simulink model "tez_model_quadcopter1"  (R2021b)
settings: Solver=VariableStepAuto  StartTime=0  StopTime=20  FixedStep=10e-3  RelTol=1e-3
values from neighbouring files (symbols this model uses):
  b = 3.59 * 10^(-5)    (= 3.59e-05)    [LQR_controller.m]
  d = 2.081 * 10^(-6)    (= 2.081e-06)    [LQR_controller.m]
  g = 9.81    [LQR_controller.m]
  Ix = 0.00963    [LQR_controller.m]
  Iy = 0.00963    [LQR_controller.m]
  Iz = 0.019    [LQR_controller.m]
  Jr = 5.225 * 10^(-5)    (= 5.225e-05)    [LQR_controller.m]
  K = lqr(A,B,Q,R)    [LQR_controller.m]
  l = 0.24    [LQR_controller.m]
  m = 0.9928    [LQR_controller.m]
undefined symbols (not defined in the file or in its folder): rad, s, sigbuilder_block
libraries: simulink_extras x5, aerolibconvert2 x4, aerolibwind2 x2, aerolibnav x2, simulink x1, sensorgpslib x1, visionsinks x1, sim3dcameralib x1, sim3dlib x1, uavsim3dlib x1
settings Model: PacingRate=1000  Creator=sevba  LastModifiedBy=SEVBAN ALTAY
settings DataIOCC: SaveFormat=StructureWithTime
settings OptimizationCC: BlockReduction=off  BufferReuse=off  ZeroExternalMemoryAtStartup=off  ZeroInternalMemoryAtStartup=off
settings DebuggingCC: AlgebraicLoopMsg=none  UnconnectedInputMsg=none  UnconnectedOutputMsg=none  UnconnectedLineMsg=none
settings RTWCC: GenCodeOnly=on  TargetLang=C++
settings GRTTargetCC: TargetLangStandard=C++11 (ISO)  CodeInterfacePackaging=C++ class
settings ExplorerConfigSet: SimMechanicsOpenEditorOnUpdate=off

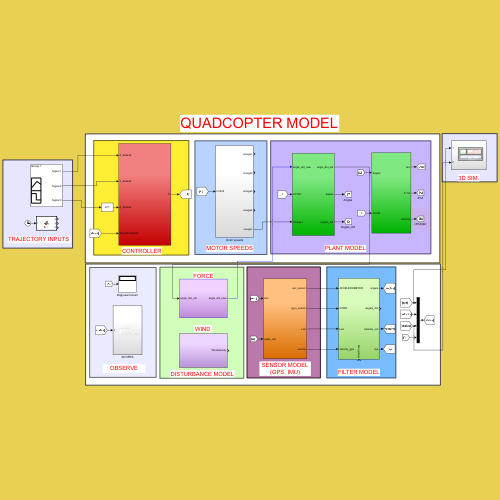
[thumbnail: Simulink's stored preview of the top-level diagram]
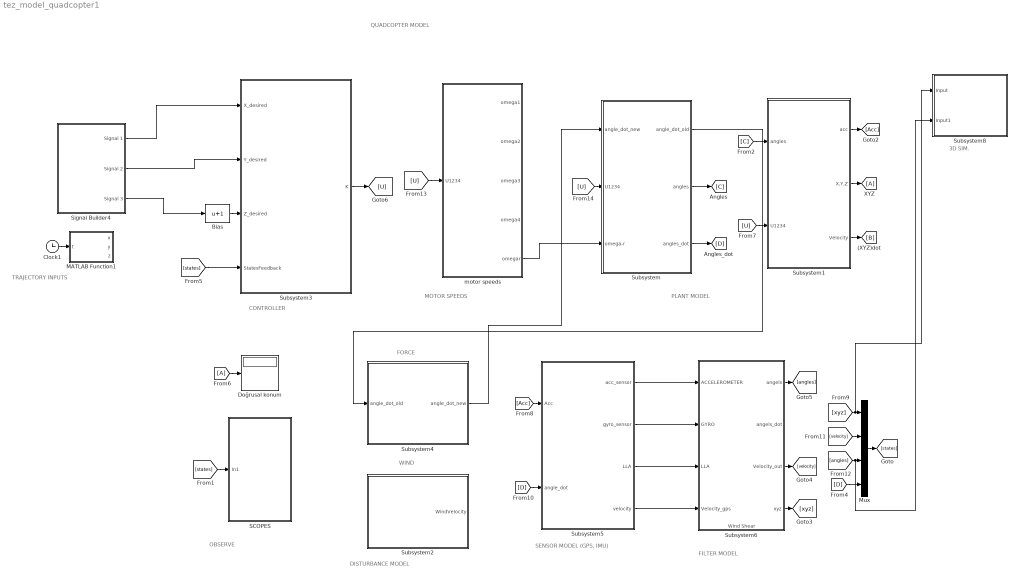
== system tez_model_quadcopter1 ==
  note: PLANT MODEL
  note: CONTROLLER
  note: MOTOR SPEEDS
  note: SENSOR MODEL
      | (GPS, IMU)
  note: FILTER MODEL
  note: DISTURBANCE MODEL
  note: OBSERVE
  note: QUADCOPTER MODEL
  note: FORCE
  note: WIND
  note: 3D SIM.
  note: TRAJECTORY INPUTS
  Bias : Bias  Bias=1
  Clock1 : Clock
  Doğrusal konum : Display
  MATLAB Function1 : MATLAB Function  TreatAsAtomicUnit=on
  Mux : Mux
  SCOPES : Subsystem
  Signal Builder4 : Subsystem  Tag=STV Subsys  LoadFcn=sigbuilder_block('load');  StartFcn=sigbuilder_block('start');  StopFcn=sigbuilder_block('stop');  ClipboardFcn=sigbuilder_block('clipboard');  mask(Sigbuilder block){tuvar=[0:10]}
      mask help: Simulink:masks:SigbuilderBlock_MD
      mask init:
      | if ~strcmp(get_param(bdroot(gcbh),'SimulationStatus'),'stopped') tuvar = sigbuilder_block('maskInit'); end
      settings: CopyFcn=sigbuilder_block('copy');  DeleteFcn=sigbuilder_block('delete');  ModelCloseFcn=sigbuilder_block('modelClose');  PreSaveFcn=sigbuilder_block('preSave');  PauseFcn=sigbuilder_block('pause');  ContinueFcn=sigbuilder_block('continue');  NameChangeFcn=sigbuilder_block('namechange');  OpenFcn=sigbuilder_block('open',[437.6 199.2 550.4 400 ]);  CloseFcn=sigbuilder_block('close');
      mask Display: plot(0, 0, 100, 100,[2, 2, 32, 32, 2], [68, 8, 8, 68, 68],[32, 2], [38, 38], [32, 19, 2],[53, 60, 44], [32, 17, 17, 2],[16, 16, 31, 31]);txt = getActiveGroup(gcbh);text(2, 100, txt,'verticalAlignment', 'top');
  Subsystem : Subsystem
  Subsystem1 : Subsystem
  Subsystem2 : Subsystem
  Subsystem3 : Subsystem
  Subsystem4 : Subsystem
  Subsystem5 : Subsystem
  Subsystem6 : Subsystem
      settings: PortSchema="{\"entries\":[{\"content\":{\"sides\":[{\"content\":{\"connectorIds\":[\"In1\",\"In2\",\"In3\",\"In4\"]},\"type\":\"ConnectorPlacement.EquallySpacedRectSide\",\"uuid\":\"cc522a2d-3ba1-4f01-ae64-adf2ce2f9772\"},{\"content\":{\"connectorIds\":[\"Out1\",\"Out2\",\"Out3\",\"Out4\"],\"side\":\"RIGHT\"},\"type\":\"ConnectorPlacement.EquallySpacedRectSide\",\"uuid\":\"95fb88f6-07dd-434c-a353-0a7a62f1e188\"},{\"content\":{\"connectorIds\":[],\"side\":\"TOP\"},\"type\":\"ConnectorPlacement.EquallySpacedRectSide\",\"uuid\":\"994d7bd2-0378-49b2-99eb-a1e64800bdf0\"},{\"content\":{\"connectorIds\":[\"In5\"],\"side\":\"BOTTOM\"},\"type\":\"ConnectorPlacement.EquallySpacedRectSide\",\"uuid\":\"a2fdffc6-4dc3-4880-acdc-0bbfa33c2e58\"}]},\"type\":\"ConnectorPlacement.EquallySpacedConnector\",\"uuid\":\"ccfbf899-2d71-4f10-9ca5-8297261b8699\"}],\"packageUris\":[\"http://schema.mathworks.com/mf0/Connector/R2020b\"],\"version\":\"1.0\"}"
  Subsystem8 : Subsystem
  motor speeds : Subsystem
  wires:
  Subsystem5/1(acc_sensor) -> Subsystem6/1(ACCELEROMETER)
  Subsystem5/2(gyro_sensor) -> Subsystem6/2(GYRO)
  Subsystem5/3(LLA) -> Subsystem6/3(LLA)
  Subsystem5/4(velocity) -> Subsystem6/4(Velocity_gps)
  [D] -> Mux/4
  Bias/1 -> Subsystem3/3(Z_desired)
  [states] -> SCOPES/1(In1)
  Mux/1 -> [states]
  [states] -> Subsystem3/4(StatesFeedback)
  [A] -> Doğrusal konum/1
  Subsystem1/1(acc) -> [Acc]
  [Acc] -> Subsystem5/1(Acc)
  Subsystem6/4(xyz) -> [xyz]
  [D] -> Subsystem5/2(angle_dot)
  Subsystem6/3(Velocity_out) -> [velocity]
  [velocity] -> Mux/2
  Subsystem6/1(angels) -> [angles]
  [angles] -> Subsystem8/2(Input1), Mux/3
  Subsystem/2(angles) -> [C]
  Subsystem/3(angles_dot) -> [D]
  [C] -> Subsystem1/1(angles)
  [U] -> motor speeds/1(U1234)
  [U] -> Subsystem1/2(U1234)
  motor speeds/5(omegar) -> Subsystem/3(omega-r)
  [U] -> Subsystem/2(U1234)
  Subsystem1/2(X,Y,Z) -> [A]
  Subsystem1/3(Velocity) -> [B]
  [xyz] -> Subsystem8/1(Input), Mux/1
  Subsystem3/1(K) -> [U]
  Clock1/1 -> MATLAB Function1/1(t)
  Subsystem4/1(angle_dot_new) -> Subsystem/1(angle_dot_new)
  Subsystem/1(angle_dot_old) -> Subsystem4/1(angle_dot_old)
  Signal Builder4/1(Signal 1) -> Subsystem3/1(X_desired)
  Signal Builder4/2(Signal 2) -> Subsystem3/2(Y_desired)
  Signal Builder4/3(Signal 3) -> Bias/1

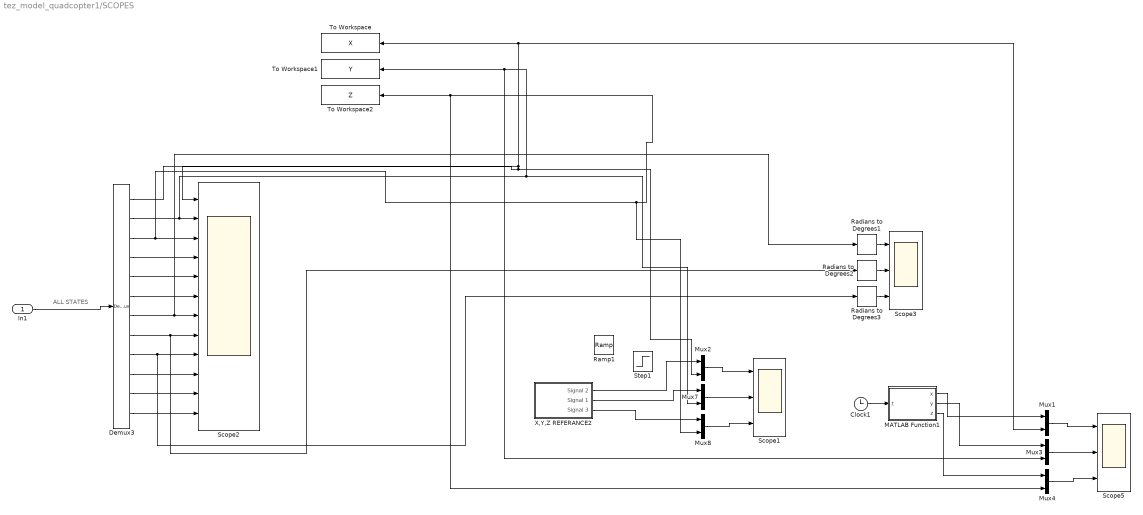
== system tez_model_quadcopter1/SCOPES ==
  note: ALL STATES
  In1 : Inport
  Clock1 : Clock
  Demux3 : Demux  Outputs=12
  MATLAB Function1 : MATLAB Function  TreatAsAtomicUnit=on
  Mux{1..4,7..8} (6 alike) : Mux  Inputs=2
  Radians to Degrees1 : simulink_extras/Transformations/Radians to Degrees
  Radians to Degrees2 : simulink_extras/Transformations/Radians to Degrees
  Radians to Degrees3 : simulink_extras/Transformations/Radians to Degrees
  Ramp1 : simulink/Sources/Ramp  slope=1  start=0  InitialOutput=0
  Scope1 : Scope  NumInputPorts=3
  Scope2 : Scope  NumInputPorts=12
  Scope3 : Scope  NumInputPorts=3
  Scope5 : Scope  NumInputPorts=3
  Step1 : Step  SampleTime=0
  To Workspace : ToWorkspace  VariableName=X  SampleTime=-1
  To Workspace1 : ToWorkspace  VariableName=Y  SampleTime=-1
  To Workspace2 : ToWorkspace  VariableName=Z  SampleTime=-1
  X,Y,Z REFERANCE2 : Subsystem  Tag=STV Subsys  LoadFcn=sigbuilder_block('load');  StartFcn=sigbuilder_block('start');  StopFcn=sigbuilder_block('stop');  ClipboardFcn=sigbuilder_block('clipboard');  mask(Sigbuilder block){tuvar=[0:10]}
      mask help: Simulink:masks:SigbuilderBlock_MD
      mask init:
      | if ~strcmp(get_param(bdroot(gcbh),'SimulationStatus'),'stopped') tuvar = sigbuilder_block('maskInit'); end
      settings: CopyFcn=sigbuilder_block('copy');  DeleteFcn=sigbuilder_block('delete');  ModelCloseFcn=sigbuilder_block('modelClose');  PreSaveFcn=sigbuilder_block('preSave');  PauseFcn=sigbuilder_block('pause');  ContinueFcn=sigbuilder_block('continue');  NameChangeFcn=sigbuilder_block('namechange');  OpenFcn=sigbuilder_block('open',[392.25 186 550.5 399.75 ]);  CloseFcn=sigbuilder_block('close');
      mask Display: plot(0, 0, 100, 100,[2, 2, 32, 32, 2], [68, 8, 8, 68, 68],[32, 2], [38, 38], [32, 19, 2],[53, 60, 44], [32, 17, 17, 2],[16, 16, 31, 31]);txt = getActiveGroup(gcbh);text(2, 100, txt,'verticalAlignment', 'top');
  wires:
  Demux3/1 -> To Workspace/1, Mux1/2, Scope2/1, Mux2/2
  Demux3/3 -> Mux8/2, Mux4/2, To Workspace2/1, Scope2/3
  Demux3/2 -> Mux7/2, Mux3/2, To Workspace1/1, Scope2/2
  Demux3/7 -> Radians to Degrees1/1, Scope2/7
  Demux3/4 -> Scope2/4
  Demux3/6 -> Scope2/6
  Demux3/10 -> Scope2/10
  Demux3/11 -> Scope2/11
  Demux3/9 -> Radians to Degrees3/1, Scope2/9
  Mux2/1 -> Scope1/1
  Mux8/1 -> Scope1/3
  Demux3/12 -> Scope2/12
  Demux3/8 -> Radians to Degrees2/1, Scope2/8
  Mux7/1 -> Scope1/2
  Radians to Degrees3/1 -> Scope3/3
  Demux3/5 -> Scope2/5
  Radians to Degrees1/1 -> Scope3/1
  Radians to Degrees2/1 -> Scope3/2
  In1/1 -> Demux3/1
  Mux3/1 -> Scope5/2
  Mux4/1 -> Scope5/3
  Mux1/1 -> Scope5/1
  Clock1/1 -> MATLAB Function1/1(t)
  MATLAB Function1/1(x) -> Mux1/1
  MATLAB Function1/3(z) -> Mux4/1
  MATLAB Function1/2(y) -> Mux3/1
  X,Y,Z REFERANCE2/1(Signal 2) -> Mux2/1
  X,Y,Z REFERANCE2/2(Signal 1) -> Mux7/1
  X,Y,Z REFERANCE2/3(Signal 3) -> Mux8/1

== system tez_model_quadcopter1/Signal Builder4 ==
  Demux : Demux  Tag=STV Demux  Outputs=3
      settings: DisplayOption=none
  FromWs : FromWorkspace  Tag=STV FromWs  VariableName=tuvar
      SigBuilderData=|
      | common.afterFinalStr = 'Extrapolate'
      | common.sampleTime = 0
      | dataSet.timeRange = [0 10]
      | dataSet.name = 'Group 1'
      | sbobj.Groups.Name = 'Group 1'
      | sbobj.Groups.Signals(1).Name = 'Signal 1'
      | sbobj.Groups.Signals(1).XData = [0 3 3 7.4 7.4 10]
      | sbobj.Groups.Signals(1).YData = [0 0 -3 -3 0 0]
      | sbobj.Groups.Signals(2).Name = 'Signal 2'
      | sbobj.Groups.Signals(2).XData = [0 1.02 1.02 6.48 6.48 10]
      | sbobj.Groups.Signals(2).YData = [0 0 1 1 0 0]
      | sbobj.Groups.Signals(3).Name = 'Signal 3'
      | sbobj.Groups.Signals(3).XData = [0 10]
      | sbobj.Groups.Signals(3).YData = [1 1]
  Signal 1 : Outport  Tag=STV Outport
  Signal 2 : Outport  Tag=STV Outport  Port=2
  Signal 3 : Outport  Tag=STV Outport  Port=3
  wires:
  Demux/1 -> Signal 1/1
  FromWs/1 -> Demux/1
  Demux/2 -> Signal 2/1
  Demux/3 -> Signal 3/1

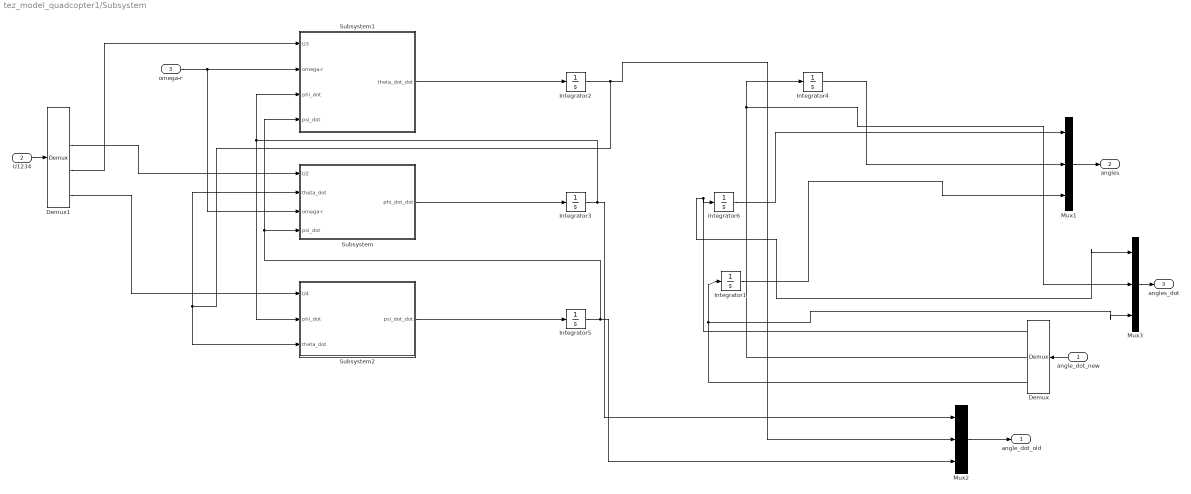
== system tez_model_quadcopter1/Subsystem ==
  angle_dot_new : Inport
  U1234 : Inport  Port=2
  omega-r : Inport  Port=3
  Demux : Demux  Outputs=3
  Demux1 : Demux
  Integrator1 : Integrator  WrapState=on
  Integrator2 : Integrator
  Integrator3 : Integrator
  Integrator4 : Integrator  WrapState=on
  Integrator5 : Integrator
  Integrator6 : Integrator  WrapState=on
  Mux1 : Mux  Inputs=3
  Mux2 : Mux  Inputs=3
  Mux3 : Mux  Inputs=3
  Subsystem : Subsystem
  Subsystem1 : Subsystem
  Subsystem2 : Subsystem
  angle_dot_old : Outport
  angles : Outport  Port=2
  angles_dot : Outport  Port=3
  wires:
  Demux1/2 -> Subsystem/1(U2)
  Integrator2/1 -> Subsystem2/3(theta_dot), Subsystem/2(theta_dot), Mux2/2
  Integrator5/1 -> Mux2/3, Subsystem1/4(psi_dot), Subsystem/4(psi_dot)
  Demux1/3 -> Subsystem1/1(U3)
  omega-r/1 -> Subsystem/3(omega-r), Subsystem1/2(omega-r)
  Demux1/4 -> Subsystem2/1(U4)
  Integrator4/1 -> Mux1/2
  Integrator6/1 -> Mux1/1
  Integrator1/1 -> Mux1/3
  Subsystem1/1(theta_dot_dot) -> Integrator2/1
  Subsystem/1(phi_dot_dot) -> Integrator3/1
  Subsystem2/1(psi_dot_dot) -> Integrator5/1
  Integrator3/1 -> Mux2/1, Subsystem1/3(phi_dot), Subsystem2/2(phi_dot)
  Demux/1 -> Mux3/1, Integrator6/1
  Demux/2 -> Integrator4/1, Mux3/2
  Demux/3 -> Integrator1/1, Mux3/3
  Mux2/1 -> angle_dot_old/1
  angle_dot_new/1 -> Demux/1
  Mux1/1 -> angles/1
  Mux3/1 -> angles_dot/1
  U1234/1 -> Demux1/1

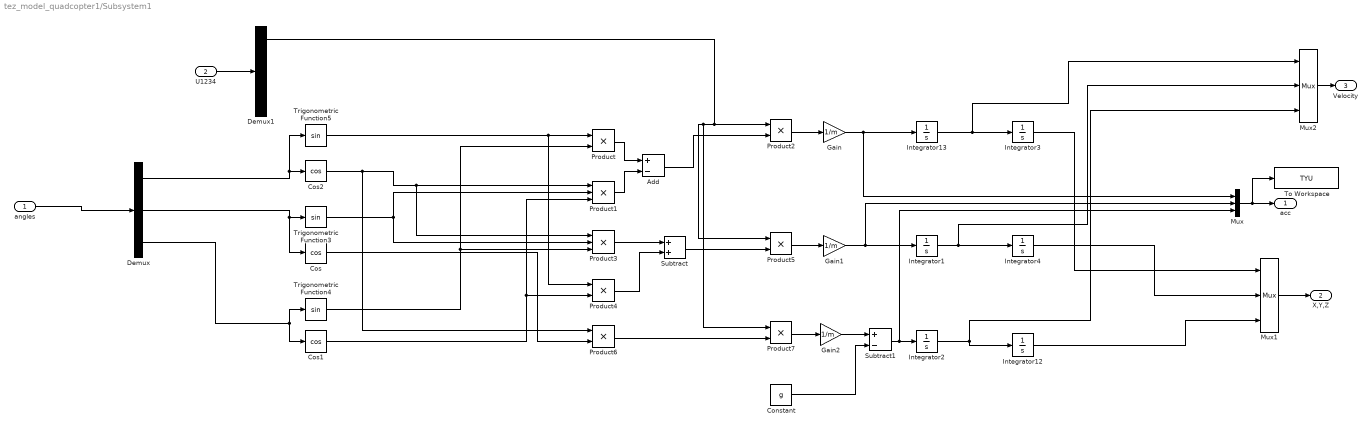
== system tez_model_quadcopter1/Subsystem1 ==
  angles : Inport
  U1234 : Inport  Port=2
  Add : Sum  Inputs=+-
  Constant : Constant  Value=g
  Cos : Trigonometry  Operator=cos
  Cos1 : Trigonometry  Operator=cos
  Cos2 : Trigonometry  Operator=cos
  Demux : Demux  Outputs=3
  Demux1 : Demux
  Gain : Gain  Gain=1/m
  Gain1 : Gain  Gain=1/m
  Gain2 : Gain  Gain=1/m
  Integrator{1..4,13} (5 alike) : Integrator
  Integrator12 : Integrator  LimitOutput=on  LowerSaturationLimit=0  WrappedStateUpperValue=100  WrappedStateLowerValue=0
  Mux : Mux  Inputs=3
  Mux1 : Mux  Inputs=3
  Mux2 : Mux  Inputs=3
  Product{,2,4..7} (6 alike) : Product
  Product1 : Product  Inputs=3
  Product3 : Product  Inputs=3
  Subtract : Sum
  Subtract1 : Sum  Inputs=+-
  To Workspace : ToWorkspace  VariableName=TYU  SampleTime=-1
  Trigonometric Function3 : Trigonometry
  Trigonometric Function4 : Trigonometry
  Trigonometric Function5 : Trigonometry
  acc : Outport
  X,Y,Z : Outport  Port=2
  Velocity : Outport  Port=3
  wires:
  Constant/1 -> Subtract1/2
  Product5/1 -> Gain1/1
  Demux/2 -> Cos/1, Trigonometric Function3/1
  Demux/1 -> Trigonometric Function5/1, Cos2/1
  Product7/1 -> Gain2/1
  Cos1/1 -> Product4/2, Product1/3
  Product3/1 -> Subtract/1
  Cos/1 -> Product6/2
  Product1/1 -> Add/2
  Product2/1 -> Gain/1
  Trigonometric Function3/1 -> Product3/2, Product1/2
  Product4/1 -> Subtract/2
  Add/1 -> Product2/2
  Subtract/1 -> Product5/2
  Trigonometric Function5/1 -> Product4/1, Product/1
  Gain1/1 -> Mux/2, Integrator1/1
  Demux/3 -> Trigonometric Function4/1, Cos1/1
  Product/1 -> Add/1
  Trigonometric Function4/1 -> Product3/3, Product/2
  Product6/1 -> Product7/2
  Cos2/1 -> Product6/1, Product1/1, Product3/1
  Integrator13/1 -> Mux2/1, Integrator3/1
  Integrator2/1 -> Mux2/3, Integrator12/1
  Gain/1 -> Mux/1, Integrator13/1
  Integrator12/1 -> Mux1/3
  Integrator4/1 -> Mux1/2
  Subtract1/1 -> Mux/3, Integrator2/1
  Demux1/1 -> Product5/1, Product7/1, Product2/1
  Gain2/1 -> Subtract1/1
  Mux/1 -> To Workspace/1, acc/1
  Integrator1/1 -> Mux2/2, Integrator4/1
  angles/1 -> Demux/1
  U1234/1 -> Demux1/1
  Mux1/1 -> X,Y,Z/1
  Integrator3/1 -> Mux1/1
  Mux2/1 -> Velocity/1

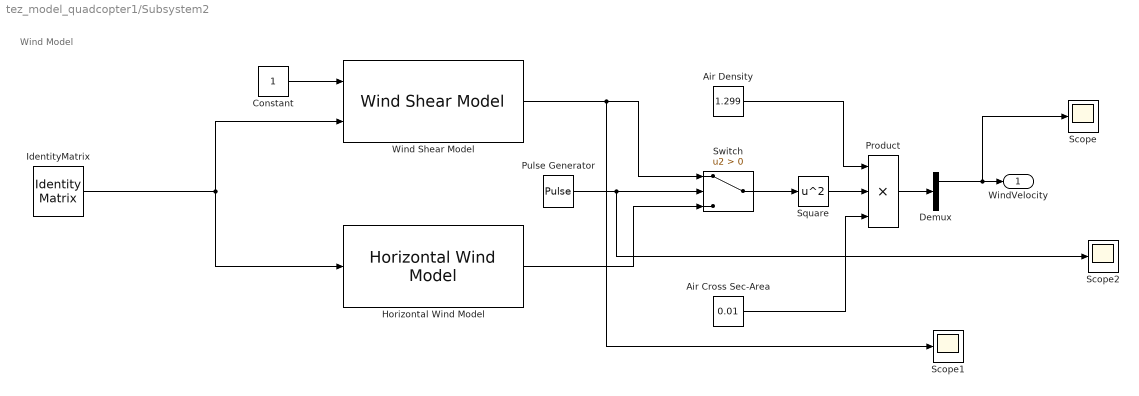
== system tez_model_quadcopter1/Subsystem2 ==
  note: Wind Model
  Air Cross Sec-Area : Constant  Value=0.01
  Air Density : Constant  Value=1.299
  Constant : Constant
  Demux : Demux  Outputs=3
  Horizontal Wind Model : aerolibwind2/Horizontal Wind Model  units=Metric (MKS)  Vw_source=Internal  Vwind=10  W_source=Internal  Wdeg=0
      settings: SourceProductBaseCode=AE
  IdentityMatrix : IdentityMatrix  OutputDimensions=3
  Product : Product  Inputs=3
  Pulse Generator : DiscretePulseGenerator  PulseType=Time based  Period=20  PulseWidth=50
  Scope : Scope
  Scope1 : Scope
  Scope2 : Scope
  Square : Math  Operator=square  SaturateOnIntegerOverflow=on
  Switch : Switch  Criteria=u2 > Threshold
  Wind Shear Model : aerolibwind2/Wind Shear Model  units=Metric (MKS)  phase=Category C - Terminal Flight Phase  W_20=10  Wdeg=0
  WindVelocity : Outport
  wires:
  Horizontal Wind Model/1 -> Switch/3
  Wind Shear Model/1 -> Scope1/1, Switch/1
  IdentityMatrix/1 -> Horizontal Wind Model/1, Wind Shear Model/2
  Square/1 -> Product/2
  Air Density/1 -> Product/1
  Air Cross Sec-Area/1 -> Product/3
  Switch/1 -> Square/1
  Pulse Generator/1 -> Scope2/1, Switch/2
  Product/1 -> Demux/1
  Demux/1 -> Scope/1, WindVelocity/1
  Constant/1 -> Wind Shear Model/1

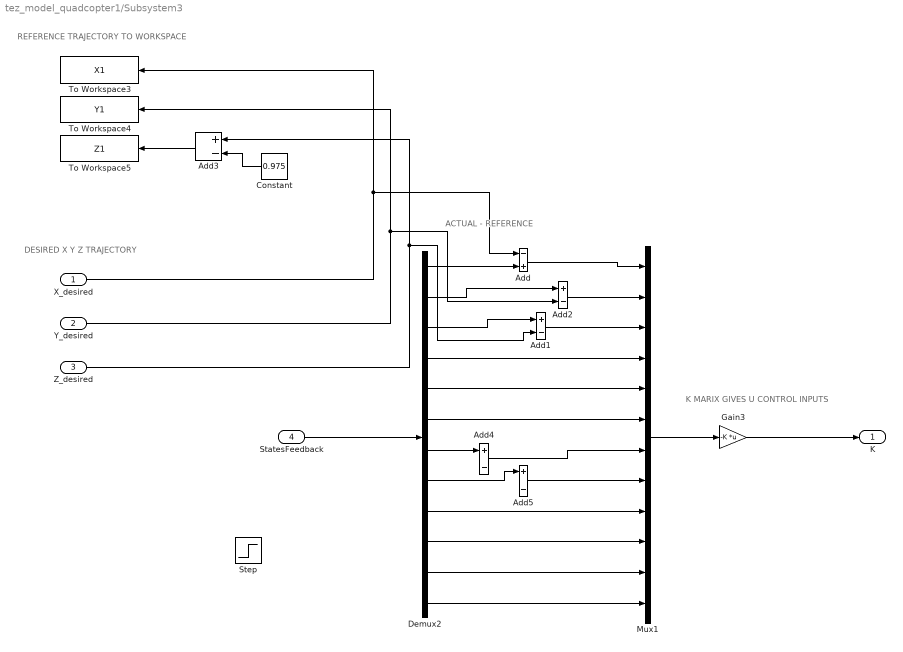
== system tez_model_quadcopter1/Subsystem3 ==
  note: K MARIX GIVES U CONTROL INPUTS
  note: ACTUAL - REFERENCE
  note: DESIRED X Y Z TRAJECTORY
  note: REFERENCE TRAJECTORY TO WORKSPACE
  X_desired : Inport
  Y_desired : Inport  Port=2
  Z_desired : Inport  Port=3
  StatesFeedback : Inport  Port=4
  Add : Sum  Inputs=-+
  Add{1..5} (5 alike) : Sum  Inputs=+-
  Constant : Constant  Value=0.975
  Demux2 : Demux  Outputs=12
  Gain3 : Gain  Gain=-K  Multiplication=Matrix(K*u)
  Mux1 : Mux  Inputs=12
  Step : Step  Time=0  SampleTime=0
  To Workspace3 : ToWorkspace  VariableName=X1  SampleTime=-1
  To Workspace4 : ToWorkspace  VariableName=Y1  SampleTime=-1
  To Workspace5 : ToWorkspace  VariableName=Z1  SampleTime=-1
  K : Outport
  wires:
  Demux2/10 -> Mux1/10
  Demux2/12 -> Mux1/12
  Add2/1 -> Mux1/2
  Demux2/11 -> Mux1/11
  Demux2/6 -> Mux1/6
  Demux2/4 -> Mux1/4
  Add/1 -> Mux1/1
  Demux2/5 -> Mux1/5
  Demux2/1 -> Add/2
  Demux2/9 -> Mux1/9
  X_desired/1 -> To Workspace3/1, Add/1
  Add1/1 -> Mux1/3
  Demux2/2 -> Add2/1
  Y_desired/1 -> To Workspace4/1, Add2/2
  Gain3/1 -> K/1
  StatesFeedback/1 -> Demux2/1
  Z_desired/1 -> Add3/1, Add1/2
  Add3/1 -> To Workspace5/1
  Constant/1 -> Add3/2
  Mux1/1 -> Gain3/1
  Demux2/3 -> Add1/1
  Demux2/7 -> Add4/1
  Add4/1 -> Mux1/7
  Demux2/8 -> Add5/1
  Add5/1 -> Mux1/8

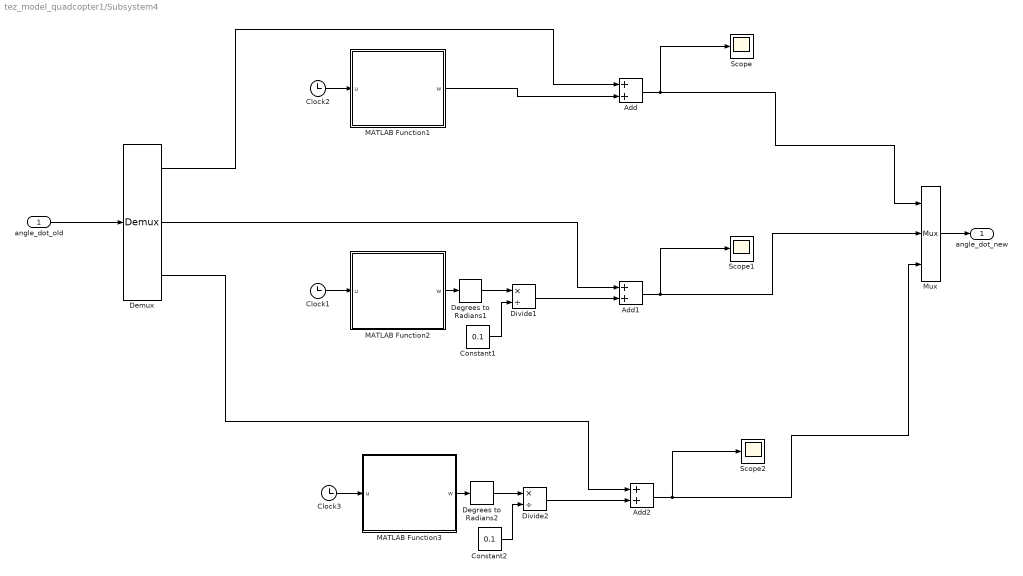
== system tez_model_quadcopter1/Subsystem4 ==
  angle_dot_old : Inport
  Add : Sum
  Add1 : Sum
  Add2 : Sum
  Clock1 : Clock
  Clock2 : Clock
  Clock3 : Clock
  Constant1 : Constant  Value=0.1
  Constant2 : Constant  Value=0.1
  Degrees to Radians1 : simulink_extras/Transformations/Degrees to Radians
  Degrees to Radians2 : simulink_extras/Transformations/Degrees to Radians
  Demux : Demux  Outputs=3
  Divide1 : Product  Inputs=*/
  Divide2 : Product  Inputs=*/
  MATLAB Function1 : MATLAB Function  TreatAsAtomicUnit=on
  MATLAB Function2 : MATLAB Function  TreatAsAtomicUnit=on
  MATLAB Function3 : MATLAB Function  TreatAsAtomicUnit=on
  Mux : Mux  Inputs=3
  Scope : Scope
  Scope1 : Scope
  Scope2 : Scope
  angle_dot_new : Outport
  wires:
  MATLAB Function1/1(w) -> Add/2
  Demux/1 -> Add/1
  Clock2/1 -> MATLAB Function1/1(u)
  Add/1 -> Scope/1, Mux/1
  Divide1/1 -> Add1/2
  Degrees to Radians1/1 -> Divide1/1
  Constant1/1 -> Divide1/2
  Add1/1 -> Scope1/1, Mux/2
  Demux/2 -> Add1/1
  MATLAB Function2/1(w) -> Degrees to Radians1/1
  Clock1/1 -> MATLAB Function2/1(u)
  MATLAB Function3/1(w) -> Degrees to Radians2/1
  Constant2/1 -> Divide2/2
  Clock3/1 -> MATLAB Function3/1(u)
  Demux/3 -> Add2/1
  Divide2/1 -> Add2/2
  Degrees to Radians2/1 -> Divide2/1
  Add2/1 -> Scope2/1, Mux/3
  Mux/1 -> angle_dot_new/1
  angle_dot_old/1 -> Demux/1

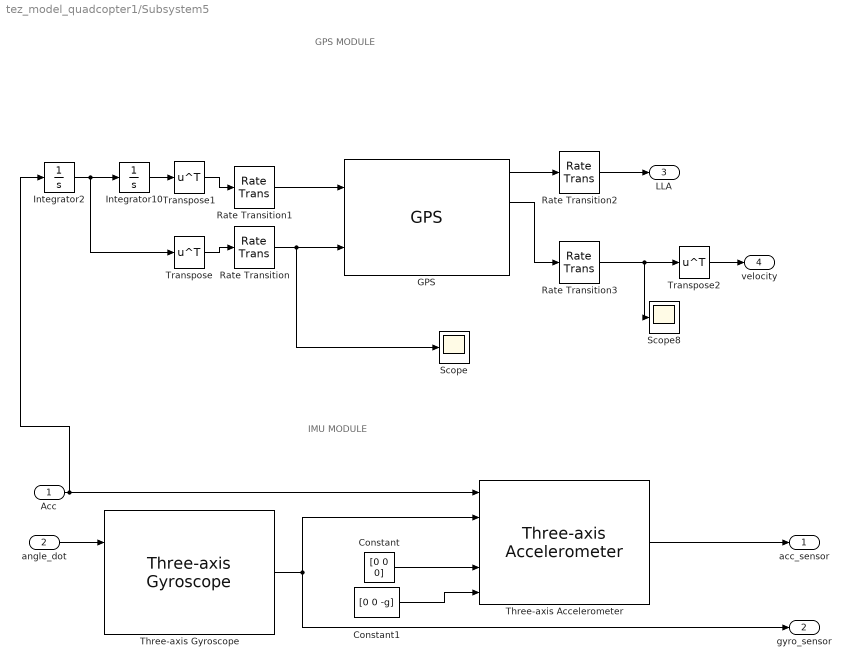
== system tez_model_quadcopter1/Subsystem5 ==
  note: IMU MODULE
  note: GPS MODULE
  Acc : Inport
  angle_dot : Inport  Port=2
  Constant : Constant  Value=[0 0 0]
  Constant1 : Constant  Value=[0 0 -g]
  GPS : sensorgpslib/GPS  DispRefFrame=NED  PositionInputFormat=Local  ReferenceLocation=[ 0, 0, 0 ]  HorizontalPositionAccuracy=0.01  VerticalPositionAccuracy=0.01  VelocityAccuracy=0.01  DecayFactor=0.999  SeedDouble=67  SimulateUsing=Interpreted execution
      settings: SourceProductBaseCode=TF,NV,UV
  Integrator10 : Integrator
  Integrator2 : Integrator
  Rate Transition : RateTransition  OutPortSampleTime=10e-3
  Rate Transition1 : RateTransition  OutPortSampleTime=10e-3
  Rate Transition2 : RateTransition  OutPortSampleTime=1/10
  Rate Transition3 : RateTransition  OutPortSampleTime=1/10
  Scope : Scope
  Scope8 : Scope
  Three-axis Accelerometer : aerolibnav/Three-axis Accelerometer  units=Metric (MKS)  acc=[0 0 0]  gtype=on  dtype_a=on  w_a=190  z_a=0.707  a_sf_cc=[1 0 0; 0 1 0; 0 0 1]  a_bias=[0 0 0]  a_Ts=10e-2  a_rand=on  a_seeds=[23093 23094 23095]  a_pow=[0.001 0.001 0.001]  a_sat="[-inf  -inf  -inf  inf inf inf]"
      settings: SourceProductBaseCode=AE
  Three-axis Gyroscope : aerolibnav/Three-axis Gyroscope  dtype_g=on  w_g=190  z_g=0.707  g_sf_cc=[1 0 0; 0 1 0; 0 0 1]  g_bias=[0 0 0]  g_sen=[0 0 0]  g_Ts=10e-2  g_rand=on  g_seeds=[23093 23094 23094]  g_pow=[0.0001 0.0001 0.000001]  g_sat="[-inf  -inf  -inf  inf inf inf]"
      settings: SourceProductBaseCode=AE
  Transpose : Math  Operator=transpose  SaturateOnIntegerOverflow=on
  Transpose1 : Math  Operator=transpose  SaturateOnIntegerOverflow=on
  Transpose2 : Math  Operator=transpose  SaturateOnIntegerOverflow=on
  acc_sensor : Outport
  gyro_sensor : Outport  Port=2
  LLA : Outport  Port=3
  velocity : Outport  Port=4
  wires:
  Constant/1 -> Three-axis Accelerometer/4
  Constant1/1 -> Three-axis Accelerometer/5
  Three-axis Gyroscope/1 -> Three-axis Accelerometer/2, gyro_sensor/1
  angle_dot/1 -> Three-axis Gyroscope/1
  Acc/1 -> Integrator2/1, Three-axis Accelerometer/1
  GPS/2 -> Rate Transition3/1
  Transpose1/1 -> Rate Transition1/1
  Integrator2/1 -> Transpose/1, Integrator10/1
  Transpose/1 -> Rate Transition/1
  Rate Transition/1 -> Scope/1, GPS/2
  Rate Transition1/1 -> GPS/1
  Integrator10/1 -> Transpose1/1
  Three-axis Accelerometer/1 -> acc_sensor/1
  Transpose2/1 -> velocity/1
  GPS/1 -> Rate Transition2/1
  Rate Transition2/1 -> LLA/1
  Rate Transition3/1 -> Scope8/1, Transpose2/1

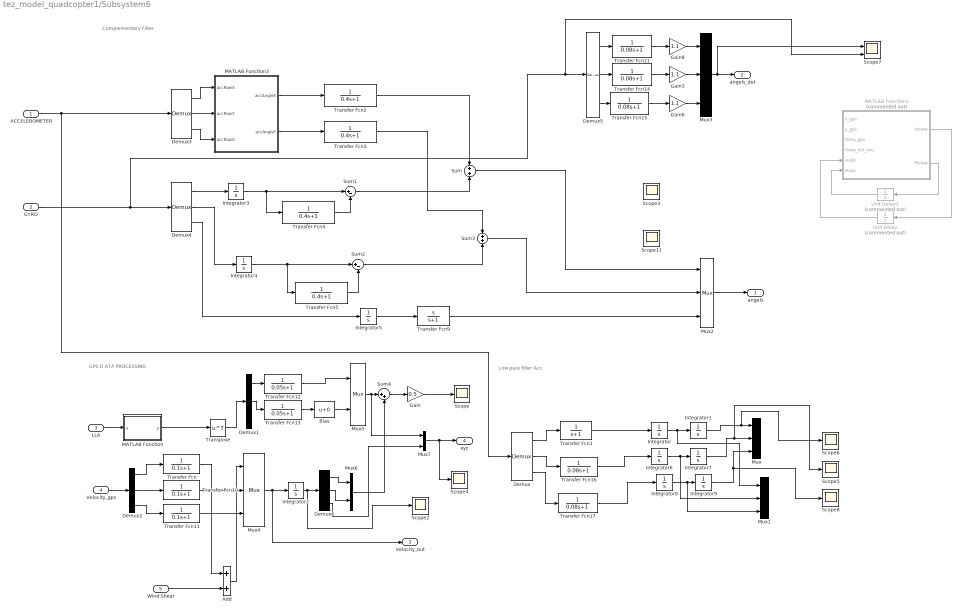
== system tez_model_quadcopter1/Subsystem6 ==
  note: GPS D ATA PROCESSING
  note: Low pass filter
      | Acc
  note: Complementary Filter
  ACCELEROMETER : Inport
  GYRO : Inport  Port=2
  LLA : Inport  Port=3
  Velocity_gps : Inport  Port=4
  Wind Shear : Inport  Port=5
  Add : Sum
  Bias : Bias
  Demux{,1..6} (7 alike) : Demux  Outputs=3
  Gain : Gain  Gain=0.5
  Gain3 : Gain  Gain=1.1
  Gain6 : Gain  Gain=1.1
  Gain8 : Gain  Gain=1.1
  Integrator{,1..9} (10 alike) : Integrator
  MATLAB Function : MATLAB Function  TreatAsAtomicUnit=on
  MATLAB Function1 : MATLAB Function  Commented=on  TreatAsAtomicUnit=on
  MATLAB Function3 : MATLAB Function  TreatAsAtomicUnit=on
  Mux{,1..4} (5 alike) : Mux  Inputs=3
  Mux5 : Mux  Inputs=2
  Mux6 : Mux  Inputs=2
  Mux7 : Mux  Inputs=2
  Scope{,2..6,8,11} (8 alike) : Scope
  Scope7 : Scope  NumInputPorts=2
  Sum : Sum
  Sum1 : Sum  Inputs=|+-
  Sum2 : Sum  Inputs=|+-
  Sum3 : Sum
  Sum4 : Sum  Inputs=|++
  Transfer Fcn : TransferFcn  Denominator=[0.1 1]
  Transfer Fcn1 : TransferFcn  Denominator=[1 1]
  Transfer Fcn10 : TransferFcn  Denominator=[0.1 1]
  Transfer Fcn11 : TransferFcn  Denominator=[0.1 1]
  Transfer Fcn12 : TransferFcn  Denominator=[0.05 1]
  Transfer Fcn13 : TransferFcn  Denominator=[0.05 1]
  Transfer Fcn14 : TransferFcn  Numerator=[1 ]  Denominator=[0.08 1]
  Transfer Fcn15 : TransferFcn  Numerator=[1 ]  Denominator=[0.08 1]
  Transfer Fcn16 : TransferFcn  Denominator=[0.08 1]
  Transfer Fcn17 : TransferFcn  Denominator=[0.08 1]
  Transfer Fcn{2..5} (4 alike) : TransferFcn  Denominator=[0.4 1]
  Transfer Fcn21 : TransferFcn  Numerator=[1 ]  Denominator=[0.08 1]
  Transfer Fcn9 : TransferFcn  Numerator=[1 0]  Denominator=[1 1]
  Transpose : Math  Operator=transpose  SaturateOnIntegerOverflow=on
  Unit Delay : UnitDelay  Commented=on  InitialCondition=[0, 0, 0.1, 1, 0.1]'  SampleTime=-1  HasFrameUpgradeWarning=on
  Unit Delay1 : UnitDelay  Commented=on  InitialCondition=diag([1000000, 1000000, 10, 10, 10],0)  SampleTime=-1  HasFrameUpgradeWarning=on
  angels : Outport
  angels_dot : Outport  Port=2
  Velocity_out : Outport  Port=3
  xyz : Outport  Port=4
  wires:
  MATLAB Function3/1(accAngleX) -> Transfer Fcn2/1
  Transfer Fcn3/1 -> Sum3/1
  Sum2/1 -> Sum3/2
  Integrator5/1 -> Transfer Fcn9/1
  Transfer Fcn2/1 -> Sum/1
  Sum1/1 -> Sum/2
  Transfer Fcn5/1 -> Sum2/2
  MATLAB Function3/2(accAngleY) -> Transfer Fcn3/1
  Demux4/2 -> Integrator4/1
  Mux2/1 -> angels/1
  Demux4/3 -> Integrator5/1
  Demux3/2 -> MATLAB Function3/2(accRawY)
  Sum/1 -> Mux2/1
  Integrator3/1 -> Sum1/1, Transfer Fcn4/1
  Demux4/1 -> Integrator3/1
  Demux3/3 -> MATLAB Function3/3(accRawZ)
  Transfer Fcn4/1 -> Sum1/2
  Demux3/1 -> MATLAB Function3/1(accRawX)
  Integrator4/1 -> Sum2/1, Transfer Fcn5/1
  ACCELEROMETER/1 -> Demux/1, Demux3/1
  Integrator/1 -> Mux1/1, Integrator1/1
  Integrator6/1 -> Mux1/2, Integrator7/1
  Integrator8/1 -> Mux1/3, Integrator9/1
  Integrator1/1 -> Scope6/1, Mux/1
  Integrator7/1 -> Scope5/1, Mux/2
  Velocity_gps/1 -> Demux2/1
  Demux2/1 -> Transfer Fcn/1
  Demux2/2 -> Transfer Fcn10/1
  Mux4/1 -> Integrator2/1, Velocity_out/1
  GYRO/1 -> Scope7/2, Demux5/1, Demux4/1
  Demux5/1 -> Transfer Fcn21/1
  Transfer Fcn21/1 -> Gain8/1
  Transfer Fcn14/1 -> Gain3/1
  Demux5/2 -> Transfer Fcn14/1
  Transfer Fcn15/1 -> Gain6/1
  Demux5/3 -> Transfer Fcn15/1
  Gain8/1 -> Mux3/1
  Gain3/1 -> Mux3/2
  Gain6/1 -> Mux3/3
  Mux3/1 -> Scope7/1, angels_dot/1
  MATLAB Function/1(y) -> Transpose/1
  LLA/1 -> MATLAB Function/1(u)
  Transpose/1 -> Demux1/1
  Demux1/1 -> Transfer Fcn12/1
  Demux1/2 -> Transfer Fcn13/1
  Transfer Fcn13/1 -> Bias/1
  Demux2/3 -> Transfer Fcn11/1
  Transfer Fcn11/1 -> Mux4/3
  Integrator2/1 -> Scope2/1, Demux6/1
  Transfer Fcn12/1 -> Mux5/1
  Mux5/1 -> Mux7/1, Sum4/1
  Demux6/2 -> Mux6/2
  Mux6/1 -> Sum4/2
  Sum4/1 -> Gain/1
  Gain/1 -> Scope/1
  Mux7/1 -> Scope4/1, xyz/1
  Demux6/3 -> Mux7/2
  Integrator9/1 -> Mux/3, Scope8/1
  Demux/1 -> Transfer Fcn1/1
  Demux/2 -> Transfer Fcn16/1
  Demux/3 -> Transfer Fcn17/1
  Transfer Fcn1/1 -> Integrator/1
  Transfer Fcn16/1 -> Integrator6/1
  Transfer Fcn17/1 -> Integrator8/1
  Demux6/1 -> Mux6/1
  MATLAB Function1/1(xknew) -> Unit Delay/1
  Unit Delay/1 -> MATLAB Function1/5(xkold)
  MATLAB Function1/2(Pknew) -> Unit Delay1/1
  Unit Delay1/1 -> MATLAB Function1/6(Pkold)
  Wind Shear/1 -> Add/2
  Transfer Fcn/1 -> Add/1
  Transfer Fcn10/1 -> Mux4/2
  Add/1 -> Mux4/1
  Sum3/1 -> Mux2/2
  Transfer Fcn9/1 -> Mux2/3
  Bias/1 -> Mux5/2

== system tez_model_quadcopter1/Subsystem8 ==
  note: Virtual Display
  note: Scene
  note: UAV
  note: Copyright 2020 The MathWorks, Inc.
  note: Sensor
  Input : Inport
  Input1 : Inport  Port=2
  Fisheye Image : visionsinks/To Video Display  windowSizeMode=Normal  openAtMdlStart=on  fullScreen=off  videoWindowX=2625  videoWindowY=376  saveWindowSize=off  videoWindowWidth=640  videoWindowHeight=640  inputColorFormat=RGB  inputType=Obsolete  imagePorts=One multidimensional signal  OutputDevice=On-screen video monitor  dataOrg=Column-major  isWindowOpen=off
  Location : Display
  Orientation : Display
  Rotation : Subsystem
  Simulation 3D Fisheye Camera : sim3dcameralib/Simulation 3D Fisheye Camera  Priority=1  sensorTag=Sim3dSensor1  sensorId=1  sensorName=Sim3dSensor1  vehTagList={'Scene Origin';'SimulinkVehicle1'}  vehTag=Scene Origin  mountLoc=Origin  offsetFlag=on  tmountOffset=[0.1, 0, 0]  extTmount=off  rmountOffset=[0, 0, 0]  extRmount=off  OpticalCenter=[640, 360]  ImageSize=[720, 1280]  RadialDistortion=[320, -0.0005, 0, 0]  StretchMatrix=[1, 0; 0, 1]  TransformOutportEnabled=on  SampleTime=-1  mountPoint=[0.1 0 0]  mountOrientation=[0 0 0]  aMode=4  ID=1
      settings: SourceProductBaseCode=AE,DR,UV,VE
  Simulation 3D Scene Configuration : sim3dlib/Simulation 3D Scene Configuration  Priority=0  ProjectFormat_internal=Default Scenes  ProjectFormat=Default Scenes  SceneDesc=US city block  ProjectName=C:\Program Files\MATLAB\R2021b\toolbox\shared\sim3d_projects\automotive_project\UE4\WindowsNoEditor\VehicleSimulation.exe  ScenePath=/Game/Maps/USCityBlock  vehTagList={'Scene Origin';'SimulinkVehicle1'}  vehTag=Scene Origin  OpVisEn=off  Ts=1/10  EnableWindow=on  EnableWeather=off  SunAltitude=40.0  SunAzimuth=90  clouds=10  wind=1  fog=0  rain=0  sensorTag=MainCamera1  sensorId=1  sensorName=MainCamera1  mountLoc=Origin  offsetFlag=off  tmountOffset=[0, 0, 0]  rmountOffset=[0, 0, 0]  HorizontalResolution=1280  VerticalResolution=720  HorizontalFOV=60  mountPoint=[0 0 0]  mountOrientation=[0 0 0]  aMode=4  ID=1
      settings: SourceProductBaseCode=AE,DR,UV,VE
  Simulation 3D UAV Vehicle : uavsim3dlib/Simulation 3D UAV Vehicle  Mesh=Quadrotor  MeshPath=/MathWorksUAVContent/UAVs/HexaRotorUAV/HexaRotor.HexaRotor  Color=Orange  ActorName=SimulinkVehicle1  InitialTranslation=[0 5 1.5]  InitialRotation=[0 0 0]  SampleTime=-1  ActorType=SimulinkVehicle  ID=1  aMode=4  ActorTag=SimulinkVehicle1
      settings: SourceProductBaseCode=UV
  Translation : Subsystem
  wires:
  Simulation 3D Fisheye Camera/2 -> Location/1
  Translation/1(Out1) -> Simulation 3D UAV Vehicle/1
  Input1/1 -> Rotation/1(Input)
  Input/1 -> Translation/1(Input)
  Simulation 3D Fisheye Camera/3 -> Orientation/1
  Rotation/1(Out1) -> Simulation 3D UAV Vehicle/2
  Simulation 3D Fisheye Camera/1 -> Fisheye Image/1

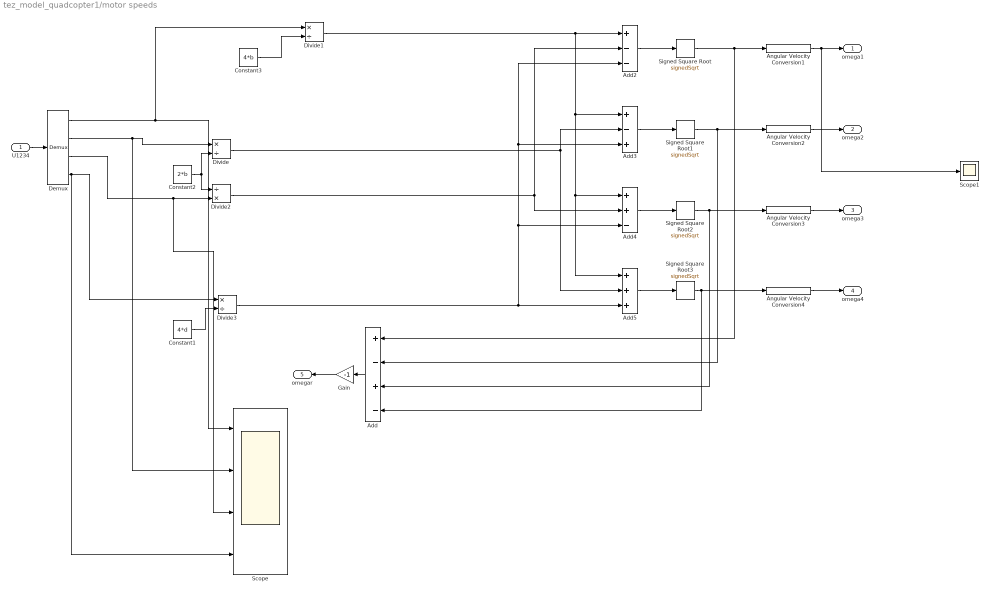
== system tez_model_quadcopter1/motor speeds ==
  U1234 : Inport
  Add : Sum  Inputs=+-+-
  Add2 : Sum  Inputs=+--
  Add3 : Sum  Inputs=+-+
  Add4 : Sum  Inputs=++-
  Add5 : Sum  Inputs=+++
  Angular Velocity Conversion{1..4} (4 alike) : aerolibconvert2/Angular Velocity Conversion  IU=rad/s  OU=rpm
  Constant1 : Constant  Value=4*d
  Constant2 : Constant  Value=2*b
  Constant3 : Constant  Value=4*b
  Demux : Demux
  Divide : Product  Inputs=*/
  Divide1 : Product  Inputs=*/
  Divide2 : Product  Inputs=/*
  Divide3 : Product  Inputs=*/
  Gain : Gain  Gain=-1
  Scope : Scope  NumInputPorts=4
  Scope1 : Scope
  Signed Square Root{,1..3} (4 alike) : Sqrt  Operator=signedSqrt  SaturateOnIntegerOverflow=on
  omega1 : Outport
  omega2 : Outport  Port=2
  omega3 : Outport  Port=3
  omega4 : Outport  Port=4
  omegar : Outport  Port=5
  wires:
  Divide3/1 -> Add4/3, Add2/3, Add3/3, Add5/3
  Divide1/1 -> Add5/1, Add4/1, Add3/1, Add2/1
  Signed Square Root3/1 -> Add/4, Angular Velocity Conversion4/1
  Signed Square Root2/1 -> Add/3, Angular Velocity Conversion3/1
  Constant1/1 -> Divide3/2
  Constant2/1 -> Divide2/1, Divide/2
  Divide2/1 -> Add2/2, Add4/2
  Add5/1 -> Signed Square Root3/1
  Angular Velocity Conversion3/1 -> omega3/1
  Divide/1 -> Add5/2, Add3/2
  Add3/1 -> Signed Square Root1/1
  Angular Velocity Conversion4/1 -> omega4/1
  Angular Velocity Conversion2/1 -> omega2/1
  Add4/1 -> Signed Square Root2/1
  Demux/3 -> Scope/3, Divide2/2
  Add2/1 -> Signed Square Root/1
  Signed Square Root/1 -> Add/1, Angular Velocity Conversion1/1
  Signed Square Root1/1 -> Add/2, Angular Velocity Conversion2/1
  Demux/2 -> Scope/2, Divide/1
  Add/1 -> Gain/1
  Gain/1 -> omegar/1
  Angular Velocity Conversion1/1 -> Scope1/1, omega1/1
  Constant3/1 -> Divide1/2
  U1234/1 -> Demux/1
  Demux/1 -> Scope/1, Divide1/1
  Demux/4 -> Scope/4, Divide3/1

== system tez_model_quadcopter1/SCOPES/X,Y,Z REFERANCE2 ==
  Demux : Demux  Tag=STV Demux  Outputs=3
      settings: DisplayOption=none
  FromWs : FromWorkspace  Tag=STV FromWs  VariableName=tuvar
      SigBuilderData=|
      | common.afterFinalStr = 'Extrapolate'
      | common.sampleTime = 0
      | dataSet.timeRange = [0 10]
      | dataSet.name = 'Group 1'
      | sbobj.Groups.Name = 'Group 1'
      | sbobj.Groups.Signals(1).Name = 'Signal 2'
      | sbobj.Groups.Signals(1).XData = [0 2.02 2.02 9 9 10]
      | sbobj.Groups.Signals(1).YData = [0 0 1 1 0 0]
      | sbobj.Groups.Signals(2).Name = 'Signal 1'
      | sbobj.Groups.Signals(2).XData = [0 5.36 5.36 10]
      | sbobj.Groups.Signals(2).YData = [0 0 1 1]
      | sbobj.Groups.Signals(3).Name = 'Signal 3'
      | sbobj.Groups.Signals(3).XData = [0 0.14 0.14 10]
      | sbobj.Groups.Signals(3).YData = [0 0 1 1]
  Signal 2 : Outport  Tag=STV Outport
  Signal 1 : Outport  Tag=STV Outport  Port=2
  Signal 3 : Outport  Tag=STV Outport  Port=3
  wires:
  FromWs/1 -> Demux/1
  Demux/1 -> Signal 2/1
  Demux/2 -> Signal 1/1
  Demux/3 -> Signal 3/1

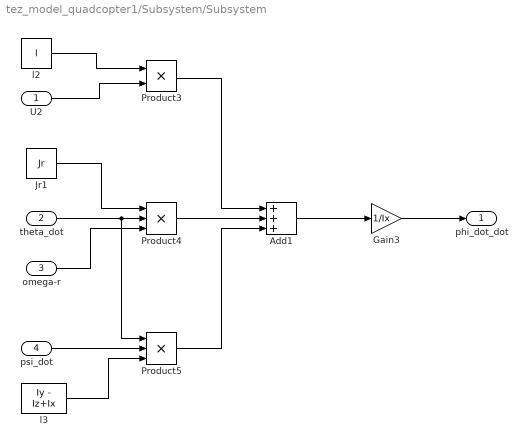
== system tez_model_quadcopter1/Subsystem/Subsystem ==
  U2 : Inport
  theta_dot : Inport  Port=2
  omega-r : Inport  Port=3
  psi_dot : Inport  Port=4
  Add1 : Sum  Inputs=+++
  Gain3 : Gain  Gain=1/Ix
  Jr1 : Constant  Value=Jr
  Product3 : Product
  Product4 : Product  Inputs=3
  Product5 : Product  Inputs=3
  l2 : Constant  Value=l
  l3 : Constant  Value=Iy - Iz+Ix
  phi_dot_dot : Outport
  wires:
  Jr1/1 -> Product4/1
  theta_dot/1 -> Product5/1, Product4/2
  psi_dot/1 -> Product5/2
  omega-r/1 -> Product4/3
  l2/1 -> Product3/1
  Product4/1 -> Add1/2
  Add1/1 -> Gain3/1
  l3/1 -> Product5/3
  Product3/1 -> Add1/1
  Product5/1 -> Add1/3
  U2/1 -> Product3/2
  Gain3/1 -> phi_dot_dot/1

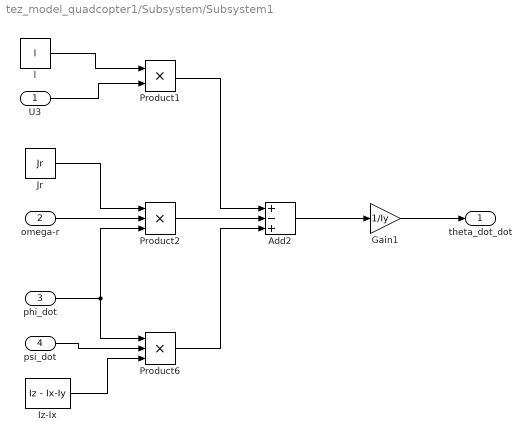
== system tez_model_quadcopter1/Subsystem/Subsystem1 ==
  U3 : Inport
  omega-r : Inport  Port=2
  phi_dot : Inport  Port=3
  psi_dot : Inport  Port=4
  Add2 : Sum  Inputs=+-+
  Gain1 : Gain  Gain=1/Iy
  Iz-Ix : Constant  Value=Iz - Ix-Iy
  Jr : Constant  Value=Jr
  Product1 : Product
  Product2 : Product  Inputs=3
  Product6 : Product  Inputs=3
  l : Constant  Value=l
  theta_dot_dot : Outport
  wires:
  l/1 -> Product1/1
  phi_dot/1 -> Product6/1, Product2/3
  omega-r/1 -> Product2/2
  Jr/1 -> Product2/1
  Iz-Ix/1 -> Product6/3
  psi_dot/1 -> Product6/2
  Product1/1 -> Add2/1
  U3/1 -> Product1/2
  Product2/1 -> Add2/2
  Gain1/1 -> theta_dot_dot/1
  Product6/1 -> Add2/3
  Add2/1 -> Gain1/1

== system tez_model_quadcopter1/Subsystem/Subsystem2 ==
  U4 : Inport
  phi_dot : Inport  Port=2
  theta_dot : Inport  Port=3
  Add1 : Sum
  Gain3 : Gain  Gain=1/Iz
  Product5 : Product  Inputs=3
  lx-Iy : Constant  Value=Iz
  psi_dot_dot : Outport
  wires:
  phi_dot/1 -> Product5/2
  Add1/1 -> Gain3/1
  lx-Iy/1 -> Product5/3
  U4/1 -> Add1/1
  Product5/1 -> Add1/2
  Gain3/1 -> psi_dot_dot/1
  theta_dot/1 -> Product5/1

== system tez_model_quadcopter1/Subsystem8/Rotation ==
  Input : Inport
  Demux : Demux  Outputs=3
  Mux : Mux  Inputs=3
  Out1 : Outport
  wires:
  Mux/1 -> Out1/1
  Input/1 -> Demux/1
  Demux/1 -> Mux/1
  Demux/2 -> Mux/2
  Demux/3 -> Mux/3

== system tez_model_quadcopter1/Subsystem8/Translation ==
  Input : Inport
  Demux : Demux  Outputs=3
  Mux : Mux  Inputs=3
  Out1 : Outport
  wires:
  Mux/1 -> Out1/1
  Demux/1 -> Mux/1
  Demux/2 -> Mux/2
  Demux/3 -> Mux/3
  Input/1 -> Demux/1

== matlab function tez_model_quadcopter1/Subsystem6/MATLAB Function3 ==
  data: accRawX input; accAngleX output; accAngleY output; accRawY input; accRawZ input
function [accAngleX, accAngleY] = fcn(accRawX, accRawY, accRawZ)

%Converting the raw accel data from g values to accel about X and Y axis

accAngleX = atan(accRawY/sqrt(power(accRawX,2) + power(accRawZ,2)));
accAngleY = atan(-1*(accRawX/sqrt(power(accRawY,2) + power(accRawZ,2))));

end

== matlab function tez_model_quadcopter1/SCOPES/MATLAB Function1 ==
  data: t input; x output; y output; z output
function [x,y,z]= fcn(t)

x = t;
y = cos(x);
z = sin(x)+1;

== matlab function tez_model_quadcopter1/Subsystem4/MATLAB Function1 ==
  data: u input; w output
function w  = fcn(u)



if (u>40 && u<40.4)
    w = 10;

else
    w=0;

end

== matlab function tez_model_quadcopter1/Subsystem6/MATLAB Function ==
  data: u input; y output
function y = fcn(u)
lla0=[0 0 0];
y=lla2ned(u,lla0,"ellipsoid");

== matlab function tez_model_quadcopter1/Subsystem6/MATLAB Function1 ==
  data: x_gps input; xknew output; y_gps input; theta_gps input; theta_dot_imu input; Pknew output; xkold input; Pkold input
function [xknew, Pknew] = EKF(x_gps, y_gps, theta_gps, theta_dot_imu, xkold, Pkold)

close all

%Sampling time T for f = 50 Hz
T = 1/50; 

%Assigning states using state vector
x = xkold(1);
y = xkold(2);
theta = xkold(3);
v = xkold(4);
theta_dot = xkold(5);


%Measurement vector [z]
z = [x_gps y_gps theta_gps theta_dot_imu]';

%Process noise covariance matrix [Q]
nu_a     = 10; %m/s^2
nu_theta = 0.1; % rad/s

%standard deviations
std_x         = 0.5* T^2 * nu_a;
std_theta     = 0.5 * T^2 * nu_theta;
std_v         = T * nu_a;
std_thetaddot = T * nu_theta; 


Q = diag([std_x^2,std_x^2, std_theta^2, std_v^2, std_thetaddot^2],0);

%Q = diag([7.6e-4,7.6e-4,5e-6,8e-2,1e-5],0);

%Sensors noise covariance matrix [R]
R = diag([3, 3, 3/500, 1/100],0);

% Measurement matrix [H]
H = [1 0 0 0 0; 0 1 0 0 0; 0 0 1 0 0; 0 0 0 0 1];

%State Transition matrix Definition ([f] non-linear matrix, [A] Jacobian linear matrix) 
model_type = 0;

if theta_dot == 0 
    model_type=1;
end

switch model_type
    case 1 % straight-line driving case   
        f =[v*cos(theta)*T + x, v*sin(theta)*T + y, theta_dot*T + theta, v, theta_dot]';

        A =[1, 0, -v*T*sin(theta), T*cos(theta), 0;
            0, 1, v*T*cos(theta), T*sin(theta), 0;
            0, 0, 1, 0, T;
            0, 0, 0, 1, 0;
            0, 0, 0, 0, 1];
        
    otherwise % non-straight line driving
        f =[v/theta_dot*(sin(theta_dot*T + theta)-sin(theta))+x, ...
            v/theta_dot*(-cos(theta_dot*T + theta)+cos(theta))+y, ...
            theta_dot*T+theta, v, theta_dot]';

        A =[1, 0, v/theta_dot*(cos(theta_dot*T + theta)-cos(theta)), ... 
            1/theta_dot*(sin(theta_dot*T + theta)-sin(theta)), ...
            v/theta_dot^2*(theta_dot*T*cos(theta_dot*T + theta) + sin(theta) - sin(theta_dot*T + theta));
            0, 1, v/theta_dot*(sin(theta_dot*T + theta)-sin(theta)), ...
            1/theta_dot*(-cos(theta_dot*T+theta)+cos(theta)), ...
            v/theta_dot^2*(theta_dot*T*sin(theta_dot*T + theta) - cos(theta) + cos(theta_dot*T + theta));
            0, 0, 1, 0, T;
            0, 0, 0, 1, 0;
            0, 0, 0, 0, 1];
end

%Prediction step
xknewp = f; 
Pknewp = A*Pkold*A'+Q;

%Estimation step
Y = z - H * xknewp;
S = H * Pknewp * H' + R;
K = Pknewp * H' /S;
xknew = xknewp + K*Y;
Pknew = Pknewp - K*H*Pknewp;
end

== matlab function tez_model_quadcopter1/Subsystem4/MATLAB Function2 ==
  data: u input; w output
function w  = fcn(u)


if (u>5.1 && u<5.2)
    w = 0;

else
    w=0;

end

== matlab function tez_model_quadcopter1/MATLAB Function1 ==
  data: t input; x output; y output; z output
function [x,y,z]= fcn(t)

x = sin(t);
y = cos(t);
z =t/4;



end

== matlab function tez_model_quadcopter1/Subsystem4/MATLAB Function3 ==
  data: u input; w output
function w  = fcn(u)



if (u>5.1 && u<5.2)
    w = 0;

else
    w=0;

end
